simulink model "solar_collector_hot_water_tank_v1"  (R2017a)
settings: Solver=VariableStepAuto  StartTime=0.0  StopTime=50000  RelTol=1e-3
values from neighbouring files (symbols this model uses):
  a1 = Ac*eta/C    (= 4.89325816065e-06)    [solar_collector_init.m]
  a2 = UL*Ac/2/C    (= 2.14080044529e-05)    [solar_collector_init.m]
  a3 = -UL*Ac/C    (= -4.28160089057e-05)    [solar_collector_init.m]
  a4 = V^-1    (= 13.3333333333)    [solar_collector_init.m]
  a5 = -a4    (= -13.3333333333)    [solar_collector_init.m]
libraries: simulink x2
settings Model: Creator=info  LastModifiedBy=admin

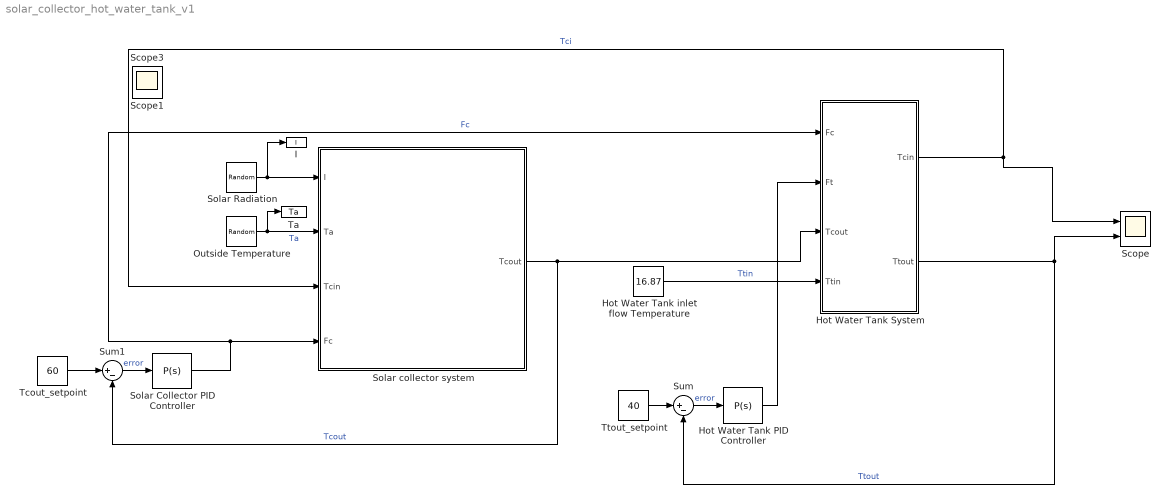
== system solar_collector_hot_water_tank_v1 ==
  Hot Water Tank PID Controller : simulink/Continuous/PID Controller  Controller=P  TimeDomain=Continuous-time  SampleTime=-1  IntegratorMethod=Forward Euler  FilterMethod=Forward Euler  Form=Parallel  UseFilter=on  ControllerParametersSource=internal  P=-0.0002  I=1.2  D=0.01  N=100  InitialConditionSource=internal  InitialConditionForIntegrator=0  InitialConditionForFilter=0  ExternalReset=none  ZeroCross=off  LimitOutput=on  UpperSaturationLimit=0.00015  LowerSaturationLimit=0  LinearizeAsGain=on  AntiWindupMode=none  Kb=1  TrackingMode=off  Kt=1  PParamMin=[]  PParamMax=[]  IParamMin=[]  IParamMax=[]  DParamMin=[]  DParamMax=[]  NParamMin=[]  NParamMax=[]  KbParamMin=[]  KbParamMax=[]  KtParamMin=[]  KtParamMax=[]  POutMin=[]  POutMax=[]  IOutMin=[]  IOutMax=[]  DOutMin=[]  DOutMax=[]  NOutMin=[]  NOutMax=[]  KbOutMin=[]  KbOutMax=[]  KtOutMin=[]  KtOutMax=[]  IntegratorOutMin=[]  IntegratorOutMax=[]  FilterOutMin=[]  FilterOutMax=[]  SumOutMin=[]  SumOutMax=[]  SumI1OutMin=[]  SumI1OutMax=[]  SumI2OutMin=[]  SumI2OutMax=[]  SumI3OutMin=[]  SumI3OutMax=[]  SumDOutMin=[]  SumDOutMax=[]  SaturationOutMin=[]  SaturationOutMax=[]  IntegratorContinuousStateAttributes=''  IntegratorStateMustResolveToSignalObject=off  IntegratorRTWStateStorageClass=Auto  FilterContinuousStateAttributes=''  FilterStateMustResolveToSignalObject=off  FilterRTWStateStorageClass=Auto  DifferentiatorICPrevScaledInput=0  DifferentiatorOutMin=[]  DifferentiatorOutMax=[]  InitialConditionSetting=State (most efficient)
  Hot Water Tank System : Subsystem
      mask Display: image('hot_water_tank.PNG');
  Hot Water Tank inlet flow Temperature : Constant  Value=16.87
  I : ToWorkspace  VariableName=I  SampleTime=-1
  Outside Temperature : RandomNumber  Mean=26  Variance=0.5  SampleTime=0.1
  Scope : Scope  NumInputPorts=2
  Solar Collector PID Controller : simulink/Continuous/PID Controller  Controller=P  TimeDomain=Continuous-time  SampleTime=-1  IntegratorMethod=Forward Euler  FilterMethod=Forward Euler  Form=Parallel  UseFilter=on  ControllerParametersSource=internal  P=-0.0002  I=1.2  D=0.01  N=100  InitialConditionSource=internal  InitialConditionForIntegrator=0  InitialConditionForFilter=0  ExternalReset=none  ZeroCross=off  LimitOutput=on  UpperSaturationLimit=0.00015  LowerSaturationLimit=0  LinearizeAsGain=on  AntiWindupMode=none  Kb=1  TrackingMode=off  Kt=1  PParamMin=[]  PParamMax=[]  IParamMin=[]  IParamMax=[]  DParamMin=[]  DParamMax=[]  NParamMin=[]  NParamMax=[]  KbParamMin=[]  KbParamMax=[]  KtParamMin=[]  KtParamMax=[]  POutMin=[]  POutMax=[]  IOutMin=[]  IOutMax=[]  DOutMin=[]  DOutMax=[]  NOutMin=[]  NOutMax=[]  KbOutMin=[]  KbOutMax=[]  KtOutMin=[]  KtOutMax=[]  IntegratorOutMin=[]  IntegratorOutMax=[]  FilterOutMin=[]  FilterOutMax=[]  SumOutMin=[]  SumOutMax=[]  SumI1OutMin=[]  SumI1OutMax=[]  SumI2OutMin=[]  SumI2OutMax=[]  SumI3OutMin=[]  SumI3OutMax=[]  SumDOutMin=[]  SumDOutMax=[]  SaturationOutMin=[]  SaturationOutMax=[]  IntegratorContinuousStateAttributes=''  IntegratorStateMustResolveToSignalObject=off  IntegratorRTWStateStorageClass=Auto  FilterContinuousStateAttributes=''  FilterStateMustResolveToSignalObject=off  FilterRTWStateStorageClass=Auto  DifferentiatorICPrevScaledInput=0  DifferentiatorOutMin=[]  DifferentiatorOutMax=[]  InitialConditionSetting=State (most efficient)
  Solar Radiation : RandomNumber  Mean=1360  Variance=0.5  SampleTime=0.1
  Solar collector system : Subsystem
      mask Display: image('collector_image.jpg');
  Sum : Sum  Inputs=|+-
  Sum1 : Sum  Inputs=|+-
  Ta : ToWorkspace  VariableName=Ta  SampleTime=-1
  Tcout_setpoint : Constant  Value=60
  Ttout_setpoint : Constant  Value=40
  Scope1 : Scope
  Scope3 : Scope
  wires:
  Hot Water Tank System/1("Tcin ") -> Scope/1, Solar collector system/3(Tcin)  "Tci"
  Outside Temperature/1 -> Ta/1, Solar collector system/2(Ta)  "Ta"
  Solar Radiation/1 -> I/1, Solar collector system/1(I)
  Hot Water Tank System/2("Ttout ") -> Sum/2, Scope/2  "Ttout"
  Ttout_setpoint/1 -> Sum/1
  Sum/1 -> Hot Water Tank PID Controller/1  "error"
  Solar Collector PID Controller/1 -> Hot Water Tank System/1("Fc "), Solar collector system/4(Fc)  "Fc"
  Hot Water Tank PID Controller/1 -> Hot Water Tank System/2(Ft)
  Hot Water Tank inlet flow Temperature/1 -> Hot Water Tank System/4("Ttin ")  "Ttin"
  Sum1/1 -> Solar Collector PID Controller/1  "error"
  Tcout_setpoint/1 -> Sum1/1
  Solar collector system/1(Tcout) -> Sum1/2, Hot Water Tank System/3("Tcout ")  "Tcout"

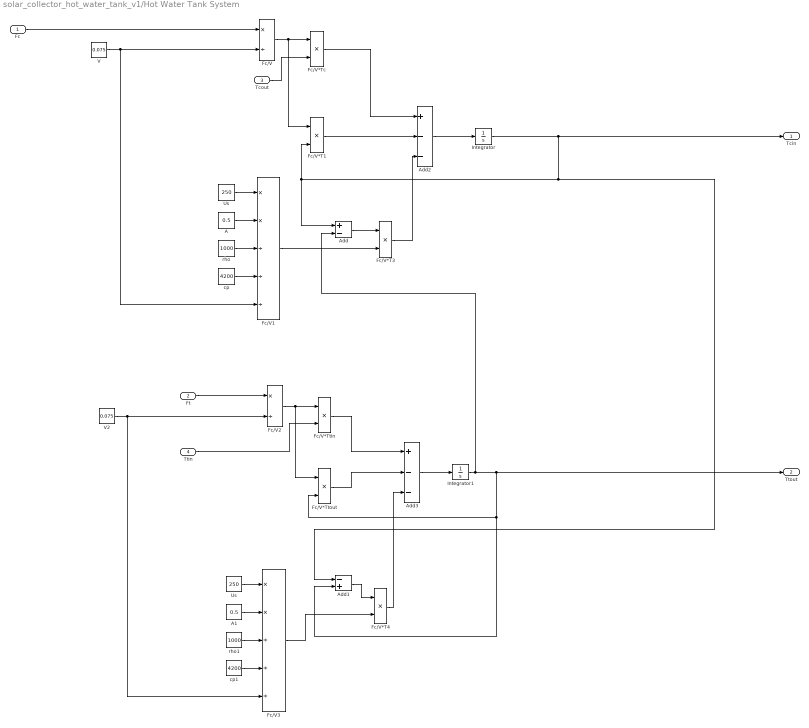
== system solar_collector_hot_water_tank_v1/Hot Water Tank System ==
  "Fc " : Inport
  Ft : Inport  Port=2
  "Tcout " : Inport  Port=3
  "Ttin " : Inport  Port=4
  A : Constant  Value=0.5
  A1 : Constant  Value=0.5
  Add : Sum  Inputs=+-
  Add1 : Sum  Inputs=-+
  Add2 : Sum  Inputs=+--
  Add3 : Sum  Inputs=+--
  Fc/V : Product  Inputs=*/
  Fc/V*T1 : Product  Inputs=**
  Fc/V*T3 : Product  Inputs=**
  Fc/V*T4 : Product  Inputs=**
  Fc/V*Tc : Product  Inputs=**
  Fc/V*Ttin : Product  Inputs=**
  Fc/V*Ttout : Product  Inputs=**
  Fc/V1 : Product  Inputs=**///
  Fc/V2 : Product  Inputs=*/
  Fc/V3 : Product  Inputs=**///
  Integrator : Integrator  InitialCondition=16.87
  Integrator1 : Integrator  InitialCondition=10
  Us : Constant  Value=250
  "Us    " : Constant  Value=250
  V : Constant  Value=0.075
  V2 : Constant  Value=0.075
  cp : Constant  Value=4200
  cp1 : Constant  Value=4200
  rho : Constant  Value=1000
  rho1 : Constant  Value=1000
  "Tcin " : Outport
  "Ttout " : Outport  Port=2
  wires:
  V/1 -> Fc/V1/5, Fc/V/2
  "Us    "/1 -> Fc/V3/1
  Integrator1/1 -> Add1/2, Fc/V*Ttout/2, "Ttout "/1, Add/2
  "Ttin "/1 -> Fc/V*Ttin/2
  "Fc "/1 -> Fc/V/1
  Fc/V/1 -> Fc/V*T1/1, Fc/V*Tc/1
  rho/1 -> Fc/V1/3
  cp1/1 -> Fc/V3/4
  A1/1 -> Fc/V3/2
  Integrator/1 -> "Tcin "/1, Add1/1, Fc/V*T1/2, Add/1
  Us/1 -> Fc/V1/1
  "Tcout "/1 -> Fc/V*Tc/2
  rho1/1 -> Fc/V3/3
  Fc/V2/1 -> Fc/V*Ttin/1, Fc/V*Ttout/1
  V2/1 -> Fc/V2/2, Fc/V3/5
  Ft/1 -> Fc/V2/1
  cp/1 -> Fc/V1/4
  A/1 -> Fc/V1/2
  Fc/V*Tc/1 -> Add2/1
  Add2/1 -> Integrator/1
  Fc/V1/1 -> Fc/V*T3/2
  Fc/V*T3/1 -> Add2/3
  Fc/V*Ttin/1 -> Add3/1
  Add3/1 -> Integrator1/1
  Add/1 -> Fc/V*T3/1
  Fc/V*T1/1 -> Add2/2
  Fc/V*Ttout/1 -> Add3/2
  Fc/V*T4/1 -> Add3/3
  Fc/V3/1 -> Fc/V*T4/2
  Add1/1 -> Fc/V*T4/1

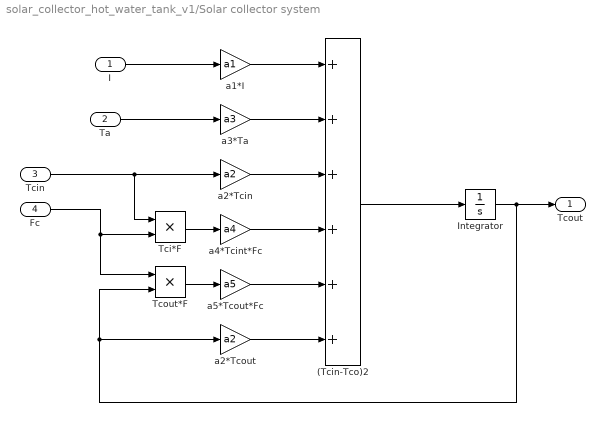
== system solar_collector_hot_water_tank_v1/Solar collector system ==
  I : Inport
  Ta : Inport  Port=2
  Tcin : Inport  Port=3
  Fc : Inport  Port=4
  (Tcin-Tco)2 : Sum  Inputs=++++++
  Integrator : Integrator  InitialCondition=10
  Tci*F : Product  Inputs=**
  Tcout*F : Product  Inputs=**
  a1*I : Gain  Gain=a1
  a2*Tcin : Gain  Gain=a2
  "a2*Tcout " : Gain  Gain=a2
  a3*Ta : Gain  Gain=a3
  a4*Tcint*Fc : Gain  Gain=a4
  "a5*Tcout*Fc " : Gain  Gain=a5
  Tcout : Outport
  wires:
  I/1 -> a1*I/1
  Integrator/1 -> "a2*Tcout "/1, Tcout*F/2, Tcout/1
  (Tcin-Tco)2/1 -> Integrator/1
  Fc/1 -> Tcout*F/1, Tci*F/2
  a1*I/1 -> (Tcin-Tco)2/1
  Ta/1 -> a3*Ta/1
  Tcin/1 -> Tci*F/1, a2*Tcin/1
  a3*Ta/1 -> (Tcin-Tco)2/2
  a2*Tcin/1 -> (Tcin-Tco)2/3
  "a5*Tcout*Fc "/1 -> (Tcin-Tco)2/5
  Tci*F/1 -> a4*Tcint*Fc/1
  a4*Tcint*Fc/1 -> (Tcin-Tco)2/4
  Tcout*F/1 -> "a5*Tcout*Fc "/1
  "a2*Tcout "/1 -> (Tcin-Tco)2/6
